simulink model "plant_model"  (R2023b)
settings: Solver=VariableStepAuto  StartTime=0.0  StopTime=10.0  RelTol=1e-3
undefined symbols (not defined in the file): param, sysc, x0
libraries: fl_lib x13, nesl_utility x7
settings Model: Creator=MPC5  LastModifiedBy=MPC5

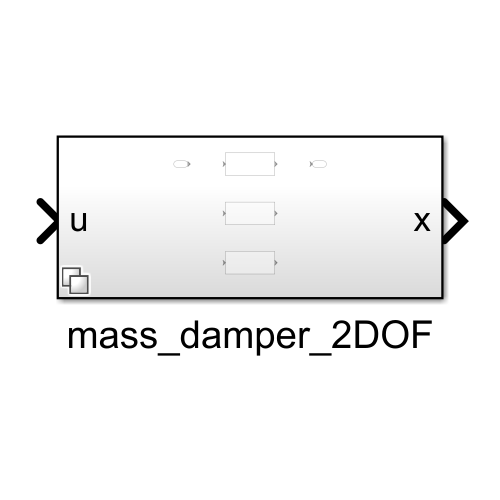
[thumbnail: Simulink's stored preview of the top-level diagram]
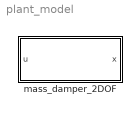
== system plant_model ==
  mass_damper_2DOF : Subsystem  Variant=on

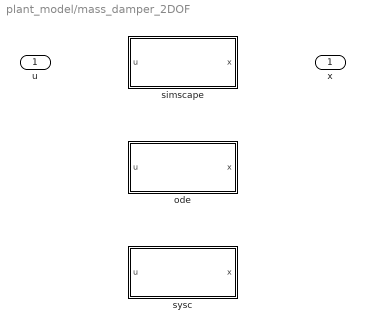
== system plant_model/mass_damper_2DOF ==
  u : Inport
  ode : Subsystem  VariantControl="plant_model_type==\"ode\""
  simscape : Subsystem  VariantControl="plant_model_type==\"simscape\""
  sysc : Subsystem  VariantControl="plant_model_type==\"sysc\""
  x : Outport

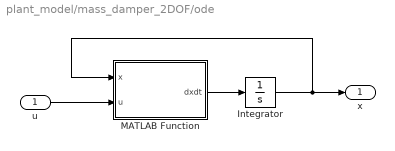
== system plant_model/mass_damper_2DOF/ode ==
  u : Inport
  Integrator : Integrator  InitialCondition=x0
  MATLAB Function : MATLAB Function  TreatAsAtomicUnit=on
  x : Outport
  wires:
  MATLAB Function/1(dxdt) -> Integrator/1
  u/1 -> MATLAB Function/2(u)
  Integrator/1 -> x/1, MATLAB Function/1(x)

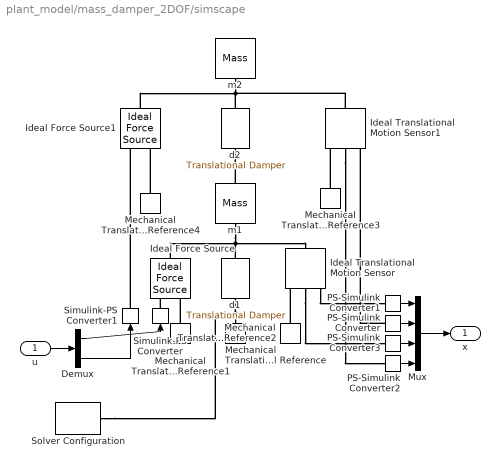
== system plant_model/mass_damper_2DOF/simscape ==
  u : Inport
  Demux : Demux  Outputs=2
  Ideal Force Source : fl_lib/Mechanical/Mechanical Sources/Ideal Force Source
  Ideal Force Source1 : fl_lib/Mechanical/Mechanical Sources/Ideal Force Source
  Ideal Translational Motion Sensor : fl_lib/Mechanical/Mechanical Sensors/Ideal Translational Motion Sensor  reference=foundation.enum.MeasurementReference.difference  acceleration_port=false  velocity_port=true  position_port=true  offset=x0(1) m
  Ideal Translational Motion Sensor1 : fl_lib/Mechanical/Mechanical Sensors/Ideal Translational Motion Sensor  reference=foundation.enum.MeasurementReference.difference  acceleration_port=false  velocity_port=true  position_port=true  offset=x0(2) m
  Mechanical Translational Reference{,1..4} (5 alike) : fl_lib/Mechanical/Translational Elements/Mechanical Translational Reference
  Mux : Mux
  PS-Simulink Converter{,1..3} (4 alike) : nesl_utility/PS-Simulink Converter  PhysicalDomain=network_engine_domain  SubClassName=ps_output  LeftPortType=input  RightPortType=output  PseudoPeriodic=off  Frequencies=[]  VectorFormat=inherit  Unit=inherit  AffineConversion=off
  Simulink-PS Converter : nesl_utility/Simulink-PS Converter  PhysicalDomain=network_engine_domain  SubClassName=ps_input  LeftPortType=input  RightPortType=output  PseudoPeriodic=off  Frequencies=[]  NoiseDistribution=none  NoiseParameters=[]  Unit=1  AffineConversion=off  FilteringAndDerivatives=provide  SimscapeFilterOrder=1  InputFilterTimeConstant=0.001  UdotUserProvided=0
  Simulink-PS Converter1 : nesl_utility/Simulink-PS Converter  PhysicalDomain=network_engine_domain  SubClassName=ps_input  LeftPortType=input  RightPortType=output  PseudoPeriodic=off  Frequencies=[]  NoiseDistribution=none  NoiseParameters=[]  Unit=1  AffineConversion=off  FilteringAndDerivatives=provide  SimscapeFilterOrder=1  InputFilterTimeConstant=0.001  UdotUserProvided=0
  Solver Configuration : nesl_utility/Solver Configuration  PhysicalDomain=network_engine_domain  SubClassName=solver  LeftPortType=input  RightPortType=generic  Tones=[]  Harmonics=[]  SimulateNoise=off  Profile=off  UseLocalSampling=off  EnableSwitchedLinearOptims=on  FrequencyDomain=off  UseCCode=off  RelTol=0.001  AbsTol=0.001  MinStep=1e-09  ToWorkspace=off  RevertToSquareIcSolve=off  NumHomotopyIterations=100  PhasorMode=off  PhasorModeNumHarmonics=1  ConsistencySolver=NEWTON_XTOL_AFTER_FTOL  IndexReductionMethod=DerivativeReplacement  DoDC=off  ResidualTolerance=1e-09  ConsistencyTolSource=GLOBAL  ConsistencyAbsTol=0.001  ConsistencyRelTol=0.001  ConsistencyTolFactor=0.001  UseLocalSolver=off  LocalSolverChoice=NE_BACKWARD_EULER_ADVANCER  ResolveIndetEquations=on  FunctionEvalNumThread=1  LocalSolverSampleTime=0.001  DoFixedCost=off  MaxNonlinIter=3  MaxModeIter=2  ComputeImpulses=off  ImpulseIterations=2  LinearAlgebra=auto  LinearAlgebraNumThread=0  EquationFormulation=NE_TIME_EF  DelaysMemoryBudget=1024  AutomaticFiltering=on  FilteringTimeConstant=0.001  PartitionStorageMethod=AS_NEEDED  PartitionMemoryBudget=1024  PartitionMethod=ROBUST  MultibodyUseLocalSolver=off  MultibodyLocalSolverChoice=ODE1  MultibodyLocalSolverSampleTime=0.001
  d1 : fl_lib/Mechanical/Translational Elements/Translational Damper  D=param.d1 N*s/m  v_specify=off  v_priority=None  v=0 m/s  v_nominal_specify=off  v_nominal_unit=m/s  v_nominal_value=1  f_specify=off  f_priority=None  f=0 N  f_nominal_specify=off  f_nominal_unit=N  f_nominal_value=1
  d2 : fl_lib/Mechanical/Translational Elements/Translational Damper  D=param.d2 N*s/m  v_specify=off  v_priority=None  v=0 m/s  v_nominal_specify=off  v_nominal_unit=m/s  v_nominal_value=1  f_specify=off  f_priority=None  f=0 N  f_nominal_specify=off  f_nominal_unit=N  f_nominal_value=1
  m1 : fl_lib/Mechanical/Translational Elements/Mass  mass=param.m1 kg  num_ports=foundation.enum.numPorts2.two  v_specify=on  v_priority=High  v=x0(3) m/s  v_nominal_specify=off  v_nominal_unit=m/s  v_nominal_value=1  f_specify=off  f_priority=None  f=0 N  f_nominal_specify=off  f_nominal_unit=N  f_nominal_value=1
      settings: InternalSimscapePortConfiguration="{\"Bottom\":[],\"Left\":[{\"id\":\"M\",\"label\":\"\",\"type\":\"foundation.mechanical.translational.translational\"}],\"Right\":[{\"id\":\"N\",\"label\":\"\",\"type\":\"foundation.mechanical.translational.translational\"}],\"Top\":[]}"
  m2 : fl_lib/Mechanical/Translational Elements/Mass  mass=param.m2 kg  num_ports=foundation.enum.numPorts2.one  v_specify=on  v_priority=High  v=x0(4) m/s  v_nominal_specify=off  v_nominal_unit=m/s  v_nominal_value=1  f_specify=off  f_priority=None  f=0 N  f_nominal_specify=off  f_nominal_unit=N  f_nominal_value=1
  x : Outport
  wires:
  PS-Simulink Converter/1 -> Mux/2
  Demux/1 -> Simulink-PS Converter/1
  PS-Simulink Converter1/1 -> Mux/1
  Mux/1 -> x/1
  u/1 -> Demux/1
  Demux/2 -> Simulink-PS Converter1/1
  PS-Simulink Converter3/1 -> Mux/3
  PS-Simulink Converter2/1 -> Mux/4
  connections:
  d1/RConn1 -- Mechanical Translational Reference/LConn1 -- Solver Configuration/RConn1
  m1/LConn1 -- d1/LConn1 -- Ideal Force Source/LConn1 -- Ideal Translational Motion Sensor/LConn1
  m2/LConn1 -- d2/LConn1 -- Ideal Force Source1/LConn1 -- Ideal Translational Motion Sensor1/LConn1
  Simulink-PS Converter/RConn1 -- Ideal Force Source/RConn1
  Ideal Translational Motion Sensor1/RConn2 -- PS-Simulink Converter2/LConn1
  Ideal Translational Motion Sensor/RConn3 -- PS-Simulink Converter1/LConn1
  Mechanical Translational Reference1/LConn1 -- Ideal Force Source/RConn2
  Ideal Translational Motion Sensor/RConn2 -- PS-Simulink Converter3/LConn1
  Mechanical Translational Reference4/LConn1 -- Ideal Force Source1/RConn2
  Mechanical Translational Reference3/LConn1 -- Ideal Translational Motion Sensor1/RConn1
  PS-Simulink Converter/LConn1 -- Ideal Translational Motion Sensor1/RConn3
  m1/RConn1 -- d2/RConn1
  Simulink-PS Converter1/RConn1 -- Ideal Force Source1/RConn1
  Mechanical Translational Reference2/LConn1 -- Ideal Translational Motion Sensor/RConn1

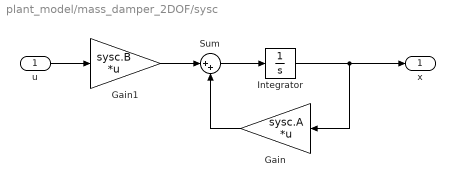
== system plant_model/mass_damper_2DOF/sysc ==
  u : Inport
  Gain : Gain  Gain=sysc.A  Multiplication=Matrix(K*u)
  Gain1 : Gain  Gain=sysc.B  Multiplication=Matrix(K*u)
  Integrator : Integrator  InitialCondition=x0
  Sum : Sum  Inputs=|++
  x : Outport
  wires:
  Sum/1 -> Integrator/1
  u/1 -> Gain1/1
  Gain1/1 -> Sum/1
  Gain/1 -> Sum/2
  Integrator/1 -> x/1, Gain/1

== matlab function plant_model/mass_damper_2DOF/ode/MATLAB Function ==
  data: x input size=param.xdim; u input size=param.udim; dxdt output size=param.xdim; param parameter
function dxdt = ode(x,u,param)
    dxdt = plant_ode(0,x,u,param);
end
